simulink model "ThreePhaseBridge"  (R2018a)
settings: Solver=VariableStepAuto  StartTime=0.0  StopTime=0.6  RelTol=1e-3  AbsTol=1e-3  EnableMultiTasking=on
values from neighbouring files (symbols this model uses):
  C2 = 1000e-6    (= 0.001)    [test_TFCheck.m]
  C2_ESL = 1e-9    (= 1e-09)    [test_TFCheck.m]
  sample_time = 1e-6    (= 1e-06)    [test_TFCheck.m]
libraries: powerlib x18
settings Model: Creator=snow_  LastModifiedBy=snow_
settings SolverCC: AutoScaleAbsTol=off
settings DataIOCC: LimitDataPoints=on  MaxDataPoints=10000
settings OptimizationCC: LifeSpan=inf
settings DebuggingCC: AllowSymbolicDim=off  SFUnexpectedBacktrackingDiag=warning  SFNoUnconditionalDefaultTransitionDiag=warning  SFExecutionAtInitializationDiag=none
settings CodeAppCC: StateflowObjectComments=on
settings GRTTargetCC: TargetLangStandard=C89/C90 (ANSI)  GeneratePreprocessorConditionals=Disable all
settings ConfigComp: CovMetricSettings=dw  CovHtmlReporting=on  CovSaveCumulativeToWorkspaceVar=on  CovSaveSingleToWorkspaceVar=on  CovExternalEMLEnable=off  CovSFcnEnable=off
settings SimscapeCC: SimscapeLogType=all  SimscapeLogDataHistory=10000

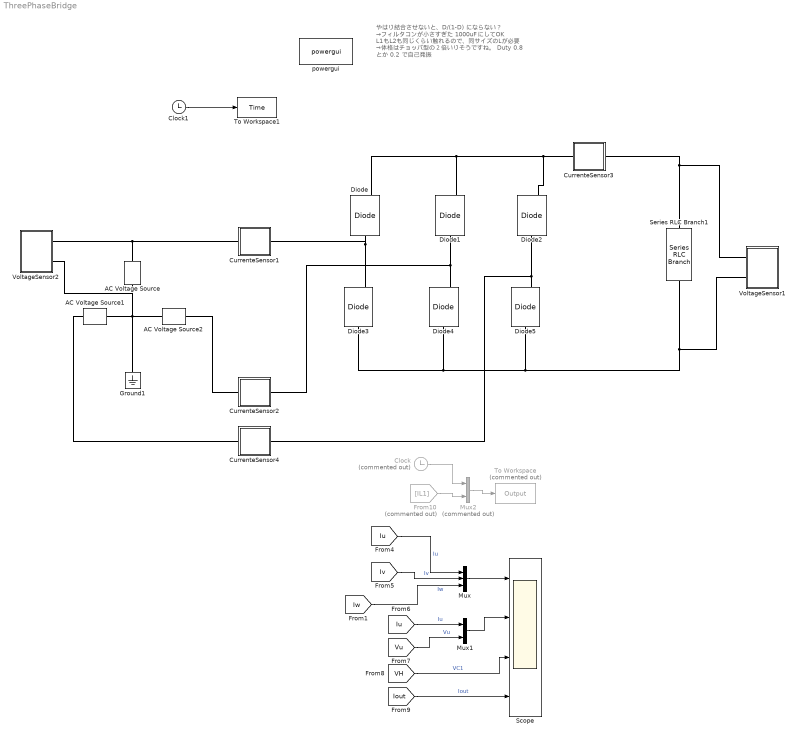
== system ThreePhaseBridge ==
  note: やはり結合させないと、D/(1-D)　にならない？
      | →フィルタコンが小さすぎた　1000uFにしてOK
      |
      | L1もL2も同じくらい触れるので、同サイズのLが必要
      | →体格はチョッパ型の２倍いりそうですね。
      |
      | Duty 0.8 とか　0.2 で自己発振
  AC Voltage Source : powerlib/Electrical Sources/AC Voltage Source  Amplitude=200  Phase=0  Frequency=60  SampleTime=0  Measurements=None  BusType=swing  Pref=10e3  Qref=0  Qmin=-inf  Qmax=+inf
      settings: AttributesFormatString=|
      | %<Amplitude> V
      | %<Frequency> Hz
  AC Voltage Source1 : powerlib/Electrical Sources/AC Voltage Source  Amplitude=200  Phase=240  Frequency=60  SampleTime=0  Measurements=None  BusType=swing  Pref=10e3  Qref=0  Qmin=-inf  Qmax=+inf
      settings: AttributesFormatString=|
      | %<Amplitude> V
      | %<Frequency> Hz
  AC Voltage Source2 : powerlib/Electrical Sources/AC Voltage Source  Amplitude=200  Phase=120  Frequency=60  SampleTime=0  Measurements=None  BusType=swing  Pref=10e3  Qref=0  Qmin=-inf  Qmax=+inf
      settings: AttributesFormatString=|
      | %<Amplitude> V
      | %<Frequency> Hz
  Clock : Clock  Commented=on
  Clock1 : Clock
  CurrenteSensor1 : Subsystem  mask{VariableName=Iu, SampleTime=1e-6}
      mask prompts: VariableName "Simulink:blkprm_prompts:ToWksVarName"
      settings: AttributesFormatString=%<VariableName>
      mask TypeOptions VariableName: To Workspace1/VariableName | Goto/GotoTag
      mask DialogControl VariableName Prompt: 変数名:
      mask Display:
      | disp("Current \n Sensor")
      | port_label('lconn', 1, '+')
      | port_label('rconn', 1, '-')
      | 
      | 
      | %set_param([gcb '/Goto'],'GotoTag',VariableName) % これは使えないっぽい
  CurrenteSensor2 : Subsystem  mask{VariableName=Iv, SampleTime=1e-6}
      mask prompts: VariableName "Simulink:blkprm_prompts:ToWksVarName"
      settings: AttributesFormatString=%<VariableName>
      mask TypeOptions VariableName: To Workspace1/VariableName | Goto/GotoTag
      mask DialogControl VariableName Prompt: 変数名:
      mask Display:
      | disp("Current \n Sensor")
      | port_label('lconn', 1, '+')
      | port_label('rconn', 1, '-')
      | 
      | 
      | %set_param([gcb '/Goto'],'GotoTag',VariableName) % これは使えないっぽい
  CurrenteSensor3 : Subsystem  mask{VariableName=Iout, SampleTime=1e-6}
      mask prompts: VariableName "Simulink:blkprm_prompts:ToWksVarName"
      settings: AttributesFormatString=%<VariableName>
      mask TypeOptions VariableName: To Workspace1/VariableName | Goto/GotoTag
      mask DialogControl VariableName Prompt: 変数名:
      mask Display:
      | disp("Current \n Sensor")
      | port_label('lconn', 1, '+')
      | port_label('rconn', 1, '-')
      | 
      | 
      | %set_param([gcb '/Goto'],'GotoTag',VariableName) % これは使えないっぽい
  CurrenteSensor4 : Subsystem  mask{VariableName=Iw, SampleTime=1e-6}
      mask prompts: VariableName "Simulink:blkprm_prompts:ToWksVarName"
      settings: AttributesFormatString=%<VariableName>
      mask TypeOptions VariableName: To Workspace1/VariableName | Goto/GotoTag
      mask DialogControl VariableName Prompt: 変数名:
      mask Display:
      | disp("Current \n Sensor")
      | port_label('lconn', 1, '+')
      | port_label('rconn', 1, '-')
      | 
      | 
      | %set_param([gcb '/Goto'],'GotoTag',VariableName) % これは使えないっぽい
  Diode{,1..5} (6 alike) : powerlib/Power Electronics/Diode  Ron=0.001  Lon=0  Vf=0.8  IC=0  UseSnubber=0  Rs=500  Cs=250e-9  Measurements=on
  From10 : From  Commented=on  GotoTag=IL1
  Ground1 : powerlib/Elements/Ground  LConnTagsString=a
  Mux : Mux  Inputs=3
  Mux1 : Mux  Inputs=2
  Mux2 : Mux  Commented=on  Inputs=2
  Scope : Scope  NumInputPorts=4
  Series RLC Branch1 : powerlib/Elements/Series RLC Branch  LConnTagsString=__new0  RConnTagsString=__new0  BranchType=R  Resistance=10  Inductance=C2_ESL  SetiL0=off  InitialCurrent=0  Capacitance=C2  Setx0=off  InitialVoltage=0  Measurements=None
      settings: AttributesFormatString=R=%<Resistance> Ohm
  To Workspace : ToWorkspace  Commented=on  VariableName=Output  SampleTime=sample_time
  To Workspace1 : ToWorkspace  VariableName=Time  SampleTime=1e-6
  VoltageSensor1 : Subsystem  mask{VariableName=VH, SampleTime=1e-6}
      mask prompts: VariableName "Simulink:blkprm_prompts:ToWksVarName"
      settings: AttributesFormatString=%<VariableName>
      mask TypeOptions VariableName: To Workspace1/VariableName | Goto/GotoTag
      mask DialogControl VariableName Prompt: 変数名:
      mask Display:
      | disp("Voltage \n Sensor")
      | port_label('lconn', 1, '+')
      | port_label('lconn', 2, '-')
      | 
      | 
      | %set_param([gcb '/Goto'],'GotoTag',VariableName) % これは使えないっぽい
  VoltageSensor2 : Subsystem  mask{VariableName=Vu, SampleTime=1e-6}
      mask prompts: VariableName "Simulink:blkprm_prompts:ToWksVarName"
      settings: AttributesFormatString=%<VariableName>
      mask TypeOptions VariableName: To Workspace1/VariableName | Goto/GotoTag
      mask DialogControl VariableName Prompt: 変数名:
      mask Display:
      | disp("Voltage \n Sensor")
      | port_label('lconn', 1, '+')
      | port_label('lconn', 2, '-')
      | 
      | 
      | %set_param([gcb '/Goto'],'GotoTag',VariableName) % これは使えないっぽい
  powergui : powerlib/powergui  Priority=1  SimulationMode=Continuous  SampleTime=50e-6  frequency=60  Iterations=50  frequencyindice=0  Pbase=100e6  ErrMax=1e-4  UnitsV=kV  UnitsW=MW  buscounter=0  FunctionMessages=off  echomessages=off  EnableUseOfTLC=off  CurrentSourceSwitches=off  DisableSnubberDevices=off  DisableRonSwitches=off  DisableVfSwitches=off  DisplayEquations=off  SolverType=Tustin/Backward Euler (TBE)  Interpol=off  ExternalGateDelay=off  methode=off  Ts=100  x0status=blocks  SPID=on  SwTol=0  HookPort=off  RestoreLinks=warning  ResistiveCurrentMeasurement=off  Frange=[0:2:500]  Ylog=off  Xlog=on  ShowGrid=off  save=off  variable=ZData  structure=0  ZoomFFT=off  StartTime=0.0  cycles=1  DisplayStyle=1  fundamental=60  FreqAxis=off  MaxFrequency=1000  frequencyindicesteady=1  RmsSteady=1  display=off
  wires:
  Mux/1 -> Scope/1
  [Iu] -> Mux/1  "Iu"
  [Iv] -> Mux/2  "Iv"
  [Iu] -> Mux1/1  "Iu"
  [Vu] -> Mux1/2  "Vu"
  Mux1/1 -> Scope/2
  [VH] -> Scope/3  "VC1"
  [Iout] -> Scope/4  "Iout"
  From10/1 -> Mux2/2
  Clock/1 -> Mux2/1
  Mux2/1 -> To Workspace/1
  Clock1/1 -> To Workspace1/1
  [Iw] -> Mux/3  "Iw"
  connections:
  Diode/RConn1 -- Diode1/RConn1 -- Diode2/RConn1 -- CurrenteSensor3/LConn1
  AC Voltage Source2/LConn1 -- VoltageSensor2/LConn2 -- AC Voltage Source/LConn1 -- Ground1/LConn1 -- AC Voltage Source1/LConn1
  Diode3/RConn1 -- CurrenteSensor1/RConn1 -- Diode/LConn1
  Diode4/RConn1 -- CurrenteSensor2/RConn1 -- Diode1/LConn1
  Diode5/RConn1 -- Diode2/LConn1 -- CurrenteSensor4/RConn1
  CurrenteSensor3/RConn1 -- VoltageSensor1/LConn1 -- Series RLC Branch1/LConn1
  Series RLC Branch1/RConn1 -- VoltageSensor1/LConn2 -- Diode5/LConn1 -- Diode4/LConn1 -- Diode3/LConn1
  AC Voltage Source/RConn1 -- VoltageSensor2/LConn1 -- CurrenteSensor1/LConn1
  AC Voltage Source2/RConn1 -- CurrenteSensor2/LConn1
  AC Voltage Source1/RConn1 -- CurrenteSensor4/LConn1

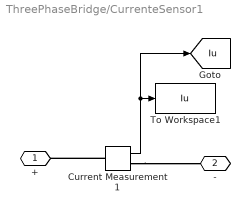
== system ThreePhaseBridge/CurrenteSensor1 ==
  Current Measurement1 : powerlib/Measurements/Current Measurement  PhasorSimulation=off  OutputType=Complex  PSBequivalent=0
  To Workspace1 : ToWorkspace  VariableName=Iu  SampleTime=SampleTime
  + : PMIOPort  Side=Left
  - : PMIOPort  Port=2  Side=Right
  tag scope: Iu=global
  wires:
  Current Measurement1/1 -> [Iu], To Workspace1/1
  connections:
  Current Measurement1/LConn1 -- +/RConn1
  Current Measurement1/RConn1 -- -/RConn1

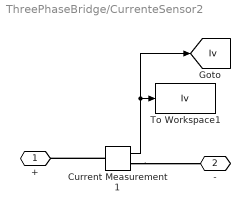
== system ThreePhaseBridge/CurrenteSensor2 ==
  Current Measurement1 : powerlib/Measurements/Current Measurement  PhasorSimulation=off  OutputType=Complex  PSBequivalent=0
  To Workspace1 : ToWorkspace  VariableName=Iv  SampleTime=SampleTime
  + : PMIOPort  Side=Left
  - : PMIOPort  Port=2  Side=Right
  tag scope: Iv=global
  wires:
  Current Measurement1/1 -> [Iv], To Workspace1/1
  connections:
  Current Measurement1/LConn1 -- +/RConn1
  Current Measurement1/RConn1 -- -/RConn1

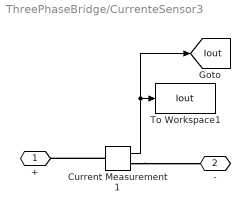
== system ThreePhaseBridge/CurrenteSensor3 ==
  Current Measurement1 : powerlib/Measurements/Current Measurement  PhasorSimulation=off  OutputType=Complex  PSBequivalent=0
  To Workspace1 : ToWorkspace  VariableName=Iout  SampleTime=SampleTime
  + : PMIOPort  Side=Left
  - : PMIOPort  Port=2  Side=Right
  tag scope: Iout=global
  wires:
  Current Measurement1/1 -> [Iout], To Workspace1/1
  connections:
  Current Measurement1/LConn1 -- +/RConn1
  Current Measurement1/RConn1 -- -/RConn1

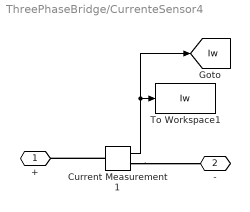
== system ThreePhaseBridge/CurrenteSensor4 ==
  Current Measurement1 : powerlib/Measurements/Current Measurement  PhasorSimulation=off  OutputType=Complex  PSBequivalent=0
  To Workspace1 : ToWorkspace  VariableName=Iw  SampleTime=SampleTime
  + : PMIOPort  Side=Left
  - : PMIOPort  Port=2  Side=Right
  tag scope: Iw=global
  wires:
  Current Measurement1/1 -> [Iw], To Workspace1/1
  connections:
  Current Measurement1/LConn1 -- +/RConn1
  Current Measurement1/RConn1 -- -/RConn1

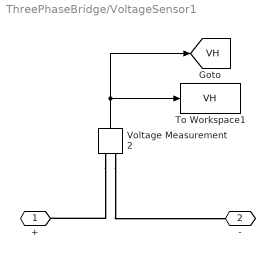
== system ThreePhaseBridge/VoltageSensor1 ==
  To Workspace1 : ToWorkspace  VariableName=VH  SampleTime=SampleTime
  Voltage Measurement2 : powerlib/Measurements/Voltage Measurement  PhasorSimulation=off  OutputType=Complex  PSBequivalent=0
  + : PMIOPort  Side=Left
  - : PMIOPort  Port=2  Side=Left
  tag scope: VH=global
  wires:
  Voltage Measurement2/1 -> [VH], To Workspace1/1
  connections:
  Voltage Measurement2/LConn1 -- +/RConn1
  Voltage Measurement2/LConn2 -- -/RConn1

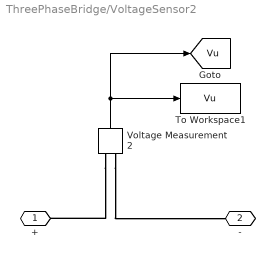
== system ThreePhaseBridge/VoltageSensor2 ==
  To Workspace1 : ToWorkspace  VariableName=Vu  SampleTime=SampleTime
  Voltage Measurement2 : powerlib/Measurements/Voltage Measurement  PhasorSimulation=off  OutputType=Complex  PSBequivalent=0
  + : PMIOPort  Side=Left
  - : PMIOPort  Port=2  Side=Left
  tag scope: Vu=global
  wires:
  Voltage Measurement2/1 -> [Vu], To Workspace1/1
  connections:
  Voltage Measurement2/LConn1 -- +/RConn1
  Voltage Measurement2/LConn2 -- -/RConn1
